simulink model "qpsk_rx_frame_sync"  (R2020a)
settings: Solver=VariableStepAuto  StartTime=0.0  StopTime=4000/3.2e6  RelTol=1e-3
PreLoadFcn:
  | setup_qpsk_receiver
InitFcn:
  | setup_qpsk_receiver
values from neighbouring files (symbols this model uses):
  tx_data = [tx_data mbuf]    [setup_receiver.m]
undefined symbols (not defined in the file or in its folder): AXI4, designMultirateFIR, Lite, xlfda_numerator
libraries: xbsIndex_r4 x244, dspmlti4 x11, hdlsllib x9, dspswit3 x4, commrandsrc3 x2, dspsigops x2, simulink x1
(part 1 of 4)
settings Model: Creator=david  LastModifiedBy=david
settings SFSimCC: CustomCodeUndefinedFunction=UseInterfaceOnly

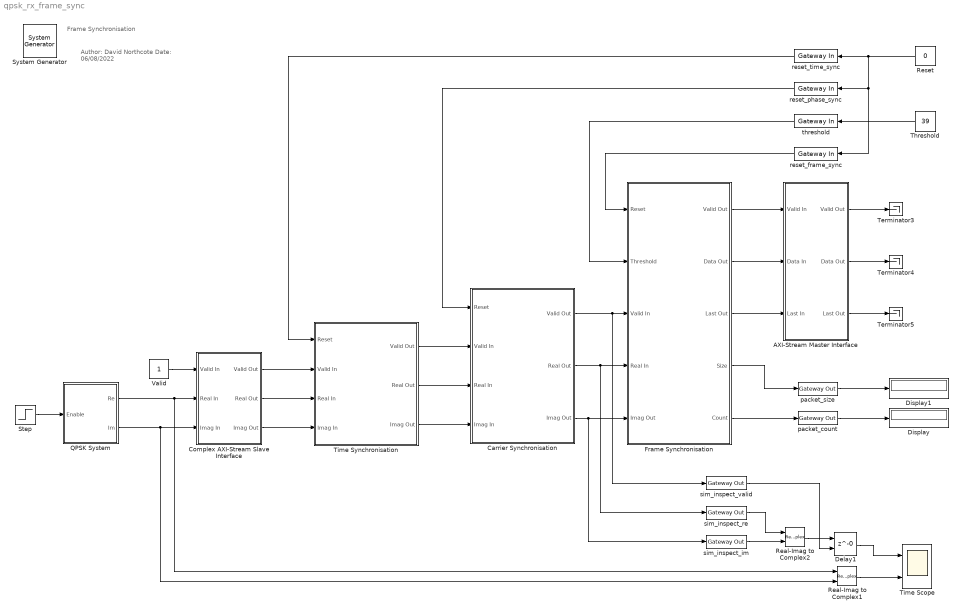
== system qpsk_rx_frame_sync ==
  note: Author: 	David Northcote
      | Date: 	06/08/2022
  note: Frame Synchronisation
  " System Generator" : xbsIndex_r4/ System Generator  Tag=genX  xilinxfamily=zynquplusRFSOC  part=xczu28dr  speed=-2-e  package=ffvg1517  synthesis_tool=Vivado  clock_wrapper=Clock Enables  directory=./netlist  proj_type=Vivado  Synth_file=Vivado Synthesis Defaults  Impl_file=Vivado Implementation Defaults  testbench=off  simulink_period=1/64e6  sysclk_period=(1/64e6)*1e9  dcm_input_clock_period=10  incr_netlist=off  trim_vbits=Everywhere in SubSystem  dbl_ovrd=According to Block Masks  core_generation=According to Block Masks  run_coregen=off  deprecated_control=off  eval_field=0  block_type=sysgen
  AXI-Stream Master Interface : Subsystem
  Carrier Synchronisation : Subsystem
  Complex AXI-Stream Slave Interface : Subsystem
  Delay1 : Delay  DelayLength=0  ShowEnablePort=on
      settings: InputPortMap=u0,e6
  Display : Display
  Display1 : Display
  Frame Synchronisation : Subsystem
  QPSK System : Subsystem
  Real-Imag to Complex1 : RealImagToComplex
  Real-Imag to Complex2 : RealImagToComplex
  Reset : Constant  Value=0  OutDataTypeStr=boolean  SampleTime=-1
  Step : Step  Time=4/12.5e3  SampleTime=1/12.5e3
  Terminator3 : Terminator
  Terminator4 : Terminator
  Terminator5 : Terminator
  Threshold : Constant  Value=39  OutDataTypeStr=uint32  SampleTime=-1
  Time Scope : Scope  NumInputPorts=2
  Time Synchronisation : Subsystem
  Valid : Constant  OutDataTypeStr=boolean  SampleTime=1/3.2e6
  packet_count : xbsIndex_r4/Gateway Out  inherit_from_input=on  hdl_port=on  rows=1  columns=1  UseAsDAC=off  DACChannel='1'  interface=AXI4-Lite  automatic_assignment=off  address_offset=24  intf_name=''  intf_description=''  timing_constraint=None  locs_specified=off  LOCs={}  io_standard={}  block_type=gatewayout
  packet_size : xbsIndex_r4/Gateway Out  inherit_from_input=on  hdl_port=on  rows=1  columns=1  UseAsDAC=off  DACChannel='1'  interface=AXI4-Lite  automatic_assignment=off  address_offset=20  intf_name=''  intf_description=''  timing_constraint=None  locs_specified=off  LOCs={}  io_standard={}  block_type=gatewayout
  reset_frame_sync : xbsIndex_r4/Gateway In  gui_display_data_type=Boolean  arith_type=Boolean  n_bits=16  bin_pt=14  preci_type=Single  exp_width=8  frac_width=24  rows=1  columns=1  quantization="Round  (unbiased: +/- Inf)"  overflow=Saturate  period=1/3.2e6  UseAsADC=off  ADCChannel='1'  interface=AXI4-Lite  automatic_assignment=off  address_offset=8  intf_name=''  intf_description=''  default_value=0  timing_constraint=None  locs_specified=off  LOCs={}  io_standard={}  inherit_from_input=off  hdl_port=on  dbl_ovrd=off  block_type=gatewayin
  reset_phase_sync : xbsIndex_r4/Gateway In  gui_display_data_type=Boolean  arith_type=Boolean  n_bits=16  bin_pt=14  preci_type=Single  exp_width=8  frac_width=24  rows=1  columns=1  quantization="Round  (unbiased: +/- Inf)"  overflow=Saturate  period=1/3.2e6  UseAsADC=off  ADCChannel='1'  interface=AXI4-Lite  automatic_assignment=off  address_offset=4  intf_name=''  intf_description=''  default_value=0  timing_constraint=None  locs_specified=off  LOCs={}  io_standard={}  inherit_from_input=off  hdl_port=on  dbl_ovrd=off  block_type=gatewayin
  reset_time_sync : xbsIndex_r4/Gateway In  gui_display_data_type=Boolean  arith_type=Boolean  n_bits=16  bin_pt=14  preci_type=Single  exp_width=8  frac_width=24  rows=1  columns=1  quantization="Round  (unbiased: +/- Inf)"  overflow=Saturate  period=1/3.2e6  UseAsADC=off  ADCChannel='1'  interface=AXI4-Lite  automatic_assignment=off  address_offset=0  intf_name=''  intf_description=''  default_value=0  timing_constraint=None  locs_specified=off  LOCs={}  io_standard={}  inherit_from_input=off  hdl_port=on  dbl_ovrd=off  block_type=gatewayin
  sim_inspect_im : xbsIndex_r4/Gateway Out  inherit_from_input=on  hdl_port=off  rows=1  columns=1  UseAsDAC=off  DACChannel='1'  interface=None  automatic_assignment=on  address_offset=hex2dec('00')  intf_name=''  intf_description=''  timing_constraint=None  locs_specified=off  LOCs={}  io_standard={}  block_type=gatewayout
  sim_inspect_re : xbsIndex_r4/Gateway Out  inherit_from_input=on  hdl_port=off  rows=1  columns=1  UseAsDAC=off  DACChannel='1'  interface=None  automatic_assignment=on  address_offset=hex2dec('00')  intf_name=''  intf_description=''  timing_constraint=None  locs_specified=off  LOCs={}  io_standard={}  block_type=gatewayout
  sim_inspect_valid : xbsIndex_r4/Gateway Out  inherit_from_input=on  hdl_port=off  rows=1  columns=1  UseAsDAC=off  DACChannel='1'  interface=None  automatic_assignment=on  address_offset=hex2dec('00')  intf_name=''  intf_description=''  timing_constraint=None  locs_specified=off  LOCs={}  io_standard={}  block_type=gatewayout
  threshold : xbsIndex_r4/Gateway In  gui_display_data_type=Fixed-point  arith_type=Unsigned  n_bits=32  bin_pt=0  preci_type=Single  exp_width=8  frac_width=24  rows=1  columns=1  quantization="Round  (unbiased: +/- Inf)"  overflow=Saturate  period=1/3.2e6  UseAsADC=off  ADCChannel='1'  interface=AXI4-Lite  automatic_assignment=off  address_offset=12  intf_name=''  intf_description=''  default_value=0  timing_constraint=None  locs_specified=off  LOCs={}  io_standard={}  inherit_from_input=off  hdl_port=on  dbl_ovrd=off  block_type=gatewayin
  wires:
  QPSK System/1(Re) -> Real-Imag to Complex1/1, Complex AXI-Stream Slave Interface/2(Real In)
  QPSK System/2(Im) -> Real-Imag to Complex1/2, Complex AXI-Stream Slave Interface/3(Imag In)
  Step/1 -> QPSK System/1(Enable)
  Valid/1 -> Complex AXI-Stream Slave Interface/1(Valid In)
  Complex AXI-Stream Slave Interface/1(Valid Out) -> Time Synchronisation/2(Valid In)
  Complex AXI-Stream Slave Interface/2(Real Out) -> Time Synchronisation/3(Real In)
  Complex AXI-Stream Slave Interface/3(Imag Out) -> Time Synchronisation/4(Imag In)
  reset_time_sync/1 -> Time Synchronisation/1(Reset)
  Reset/1 -> reset_phase_sync/1, reset_frame_sync/1, reset_time_sync/1
  Time Synchronisation/1(Valid Out) -> Carrier Synchronisation/2(Valid In)
  Time Synchronisation/2(Real Out) -> Carrier Synchronisation/3(Real In)
  Time Synchronisation/3(Imag Out) -> Carrier Synchronisation/4(Imag In)
  reset_phase_sync/1 -> Carrier Synchronisation/1(Reset)
  Carrier Synchronisation/2(Real Out) -> sim_inspect_re/1, Frame Synchronisation/4(Real In)
  Carrier Synchronisation/1(Valid Out) -> sim_inspect_valid/1, Frame Synchronisation/3(Valid In)
  threshold/1 -> Frame Synchronisation/2(Threshold)
  reset_frame_sync/1 -> Frame Synchronisation/1(Reset)
  Threshold/1 -> threshold/1
  Carrier Synchronisation/3(Imag Out) -> Frame Synchronisation/5(Imag Out), sim_inspect_im/1
  Frame Synchronisation/5(Count) -> packet_count/1
  Frame Synchronisation/4(Size) -> packet_size/1
  AXI-Stream Master Interface/1(Valid Out) -> Terminator3/1
  AXI-Stream Master Interface/2(Data Out) -> Terminator4/1
  AXI-Stream Master Interface/3(Last Out) -> Terminator5/1
  Real-Imag to Complex1/1 -> Time Scope/2
  sim_inspect_valid/1 -> Delay1/2
  Real-Imag to Complex2/1 -> Delay1/1
  sim_inspect_re/1 -> Real-Imag to Complex2/1
  sim_inspect_im/1 -> Real-Imag to Complex2/2
  Delay1/1 -> Time Scope/1
  Frame Synchronisation/1(Valid Out) -> AXI-Stream Master Interface/1(Valid In)
  Frame Synchronisation/2(Data Out) -> AXI-Stream Master Interface/2(Data In)
  Frame Synchronisation/3(Last Out) -> AXI-Stream Master Interface/3(Last In)
  packet_count/1 -> Display/1
  packet_size/1 -> Display1/1

== system qpsk_rx_frame_sync/AXI-Stream Master Interface ==
  note: AXI-Stream
  Valid In : Inport
  Data In : Inport  Port=2
  Last In : Inport  Port=3
  m_axis_tdata : xbsIndex_r4/Gateway Out  inherit_from_input=off  hdl_port=on  rows=1  columns=1  UseAsDAC=off  DACChannel='1'  interface=None  automatic_assignment=on  address_offset=hex2dec('00')  intf_name=''  intf_description=''  timing_constraint=None  locs_specified=off  LOCs={}  io_standard={}  block_type=gatewayout
  m_axis_tlast : xbsIndex_r4/Gateway Out  inherit_from_input=off  hdl_port=on  rows=1  columns=1  UseAsDAC=off  DACChannel='1'  interface=None  automatic_assignment=on  address_offset=hex2dec('00')  intf_name=''  intf_description=''  timing_constraint=None  locs_specified=off  LOCs={}  io_standard={}  block_type=gatewayout
  m_axis_tvalid : xbsIndex_r4/Gateway Out  inherit_from_input=off  hdl_port=on  rows=1  columns=1  UseAsDAC=off  DACChannel='1'  interface=None  automatic_assignment=on  address_offset=hex2dec('00')  intf_name=''  intf_description=''  timing_constraint=None  locs_specified=off  LOCs={}  io_standard={}  block_type=gatewayout
  Valid Out : Outport  VectorParamsAs1DForOutWhenUnconnected=off
  Data Out : Outport  Port=2  VectorParamsAs1DForOutWhenUnconnected=off
  Last Out : Outport  Port=3  VectorParamsAs1DForOutWhenUnconnected=off
  wires:
  Data In/1 -> m_axis_tdata/1
  Valid In/1 -> m_axis_tvalid/1
  m_axis_tdata/1 -> Data Out/1
  m_axis_tvalid/1 -> Valid Out/1
  Last In/1 -> m_axis_tlast/1
  m_axis_tlast/1 -> Last Out/1

== system qpsk_rx_frame_sync/Carrier Synchronisation ==
  Reset : Inport
  Valid In : Inport  Port=2
  Real In : Inport  Port=3
  Imag In : Inport  Port=4
  Convert : xbsIndex_r4/Convert  gui_display_data_type=Fixed-point  arith_type="Signed  (2's comp)"  n_bits=16  bin_pt=14  float_type=Single  exp_bits=8  fraction_bits=24  quantization=Truncate  overflow=Wrap  en=off  latency=0  pipeline=off  dbl_ovrd=off  block_type=convert
  Convert1 : xbsIndex_r4/Convert  gui_display_data_type=Fixed-point  arith_type="Signed  (2's comp)"  n_bits=16  bin_pt=14  float_type=Single  exp_bits=8  fraction_bits=24  quantization=Truncate  overflow=Wrap  en=off  latency=0  pipeline=off  dbl_ovrd=off  block_type=convert
  De-Rotate Constellation : Subsystem
  Generate Angle Error : Subsystem
  Generate NCO : Subsystem
  Valid Out : Outport  VectorParamsAs1DForOutWhenUnconnected=off
  Real Out : Outport  Port=2  VectorParamsAs1DForOutWhenUnconnected=off
  Imag Out : Outport  Port=3  VectorParamsAs1DForOutWhenUnconnected=off
  wires:
  Reset/1 -> Generate NCO/3(Reset)
  De-Rotate Constellation/1(Imag Out) -> Convert/1
  De-Rotate Constellation/2(Real Out) -> Convert1/1
  De-Rotate Constellation/3(Valid Out) -> Valid Out/1, Generate Angle Error/3(Valid In)
  Generate NCO/3(Valid Out) -> De-Rotate Constellation/6(Valid Error)
  Generate NCO/2(Real Out) -> De-Rotate Constellation/5(Real Error)
  Generate NCO/1(Imag Out) -> De-Rotate Constellation/4(Imag Error)
  Generate Angle Error/1(Angle) -> Generate NCO/1(Angle)
  Generate Angle Error/2(Valid Out) -> Generate NCO/2(Valid In)
  Valid In/1 -> De-Rotate Constellation/3(Valid In)
  Real In/1 -> De-Rotate Constellation/2(Real In)
  Imag In/1 -> De-Rotate Constellation/1(Imag In)
  Convert/1 -> Imag Out/1, Generate Angle Error/1(Imag In)
  Convert1/1 -> Real Out/1, Generate Angle Error/2(Real In)

== system qpsk_rx_frame_sync/Complex AXI-Stream Slave Interface ==
  note: AXI-Stream Real
  note: AXI-Stream Imag
  Valid In : Inport
  Real In : Inport  Port=2
  Imag In : Inport  Port=3
  Terminator : Terminator
  s_axis_tdata_im : xbsIndex_r4/Gateway In  gui_display_data_type=Fixed-point  arith_type="Signed  (2's comp)"  n_bits=16  bin_pt=14  preci_type=Single  exp_width=8  frac_width=24  rows=1  columns=1  quantization="Round  (unbiased: +/- Inf)"  overflow=Saturate  period=1/3.2e6  UseAsADC=off  ADCChannel='1'  interface=None  automatic_assignment=on  address_offset=hex2dec('00')  intf_name=''  intf_description=''  default_value=0  timing_constraint=None  locs_specified=off  LOCs={}  io_standard={}  inherit_from_input=off  hdl_port=on  dbl_ovrd=off  block_type=gatewayin
  s_axis_tdata_re : xbsIndex_r4/Gateway In  gui_display_data_type=Fixed-point  arith_type="Signed  (2's comp)"  n_bits=16  bin_pt=14  preci_type=Single  exp_width=8  frac_width=24  rows=1  columns=1  quantization="Round  (unbiased: +/- Inf)"  overflow=Saturate  period=1/3.2e6  UseAsADC=off  ADCChannel='1'  interface=None  automatic_assignment=on  address_offset=hex2dec('00')  intf_name=''  intf_description=''  default_value=0  timing_constraint=None  locs_specified=off  LOCs={}  io_standard={}  inherit_from_input=off  hdl_port=on  dbl_ovrd=off  block_type=gatewayin
  s_axis_tvalid_im : xbsIndex_r4/Gateway In  gui_display_data_type=Boolean  arith_type=Boolean  n_bits=16  bin_pt=14  preci_type=Single  exp_width=8  frac_width=24  rows=1  columns=1  quantization="Round  (unbiased: +/- Inf)"  overflow=Saturate  period=1/3.2e6  UseAsADC=off  ADCChannel='1'  interface=None  automatic_assignment=on  address_offset=hex2dec('00')  intf_name=''  intf_description=''  default_value=0  timing_constraint=None  locs_specified=off  LOCs={}  io_standard={}  inherit_from_input=off  hdl_port=on  dbl_ovrd=off  block_type=gatewayin
  s_axis_tvalid_re : xbsIndex_r4/Gateway In  gui_display_data_type=Boolean  arith_type=Boolean  n_bits=16  bin_pt=14  preci_type=Single  exp_width=8  frac_width=24  rows=1  columns=1  quantization="Round  (unbiased: +/- Inf)"  overflow=Saturate  period=1/3.2e6  UseAsADC=off  ADCChannel='1'  interface=None  automatic_assignment=on  address_offset=hex2dec('00')  intf_name=''  intf_description=''  default_value=0  timing_constraint=None  locs_specified=off  LOCs={}  io_standard={}  inherit_from_input=off  hdl_port=on  dbl_ovrd=off  block_type=gatewayin
  Valid Out : Outport  VectorParamsAs1DForOutWhenUnconnected=off
  Real Out : Outport  Port=2  VectorParamsAs1DForOutWhenUnconnected=off
  Imag Out : Outport  Port=3  VectorParamsAs1DForOutWhenUnconnected=off
  wires:
  Imag In/1 -> s_axis_tdata_im/1
  s_axis_tdata_re/1 -> Real Out/1
  s_axis_tdata_im/1 -> Imag Out/1
  Valid In/1 -> s_axis_tvalid_im/1, s_axis_tvalid_re/1
  s_axis_tvalid_re/1 -> Valid Out/1
  s_axis_tvalid_im/1 -> Terminator/1
  Real In/1 -> s_axis_tdata_re/1

== system qpsk_rx_frame_sync/Frame Synchronisation ==
  Reset : Inport
  Threshold : Inport  Port=2
  Valid In : Inport  Port=3
  Real In : Inport  Port=4
  Imag Out : Inport  Port=5
  Convert to AXI-Stream : Subsystem
  Frame Sync : Subsystem
  Valid Out : Outport  VectorParamsAs1DForOutWhenUnconnected=off
  Data Out : Outport  Port=2  VectorParamsAs1DForOutWhenUnconnected=off
  Last Out : Outport  Port=3  VectorParamsAs1DForOutWhenUnconnected=off
  Size : Outport  Port=4  VectorParamsAs1DForOutWhenUnconnected=off
  Count : Outport  Port=5  VectorParamsAs1DForOutWhenUnconnected=off
  wires:
  Convert to AXI-Stream/4(Size) -> Size/1
  Frame Sync/3(count) -> Count/1
  Convert to AXI-Stream/5(Reset) -> Frame Sync/6(Reset)
  Convert to AXI-Stream/3(Last Out) -> Last Out/1
  Convert to AXI-Stream/2(Valid Out) -> Valid Out/1
  Convert to AXI-Stream/1(Data Out) -> Data Out/1
  Frame Sync/2(Valid Out) -> Convert to AXI-Stream/2(Valid In)
  Frame Sync/1(Data Out) -> Convert to AXI-Stream/1(Data In)
  Reset/1 -> Frame Sync/5(reset_count)
  Valid In/1 -> Frame Sync/4(Valid In)
  Real In/1 -> Frame Sync/2(Real)
  Threshold/1 -> Frame Sync/1(Threshold)
  Imag Out/1 -> Frame Sync/3(Imag)

== system qpsk_rx_frame_sync/QPSK System ==
  Enable : Inport
  Complex to Real-Imag : ComplexToRealImag
  QPSK RX Generation : Subsystem
  QPSK TX Generation : Subsystem
  RF Balun Gain RX : Gain  Gain=1/2
  RF Balun Gain TX : Gain  Gain=1/2
  RF-ADC : Subsystem  mask{fs_ghz=1.024, decim=8x, ssr=2, mode=Fine, fc=0.064, fph=0, fcoarse=fs/4}
      mask prompts: fs_ghz "Sample Rate (GHz):"; decim "Interpolation Mode:"; ssr "Samples per AXI4-Stream Cycle:"; mode "Mixer Type:"; fc "NCO Frequency (GHz):"; fph "NCO Phase (Rads):"; fcoarse "Frequency:"
      mask init:
      | % Obtain the sample rate in Hz
      | fs = str2double(get_param(gcb, 'fs_ghz'))*1e9;
      | 
      | % Set the mode of the RF-DAC interpolation filter
      | switch get_param(gcb, 'decim')
      |     case '1x'
      |         D = 1;
      |     case '2x'
      |         D = 2;
      |     case '4x'
      |         D = 4;
      |     case '8x'
      |         D = 8;
      |     otherwise
      |         D = 1;
      | end
      | 
      | % Get the AXI-Stream clock for display to user
      | axi_clk = (fs/(str2double(get_param(gcb, 'ssr'))*D))*1e-6;
      | 
      | % Get the block mask object to manipulate settings
      | mo = get_param(gcb, 'MaskObject');
      | 
      | % Update text to display the required AXI-Stream clock
      | tc = mo.getDialogControl('axi_text');
      | tc.Prompt = ['      Required AXI-Stream Clock: ', num2str(axi_clk), ' MHz'];
      | 
      | % Set the RF-DAC Mixer mode
      | switch get_param(gcb, 'mode')
      |     case 'Bypass'
      |         m = 0;
      |     case 'Coarse'
      |         m = 1;
      |     case 'Fine'
      |         m = 2;
      |     otherwise
      |         m = 0;
      | end
      | 
      | % Set the RF-DAC Coarse Mixer mode
      | switch get_param(gcb, 'fcoarse')
      |     case 'fs/2'
      |         mc = 0;
      |     case 'fs/4'
      |         mc = 1;
      |     case '-fs/4'
      |         mc = 2;
      |     otherwise
      |         mc = 0;
      | end
      | 
      | % Set other blocks
      | set_param([gcb, '/Decimation Filter'], 'decim', get_param(gcb, 'decim'));
      mask Callback fs_ghz:
      | % Obtain the sample rate in Hz
      | fs = str2double(get_param(gcb, 'fs_ghz'))*1e9;
      | 
      | % Set the mode of the RF-DAC interpolation filter
      | switch get_param(gcb, 'decim')
      |     case '1x'
      |         D = 1;
      |     case '2x'
      |         D = 2;
      |     case '4x'
      |         D = 4;
      |     case '8x'
      |         D = 8;
      |     otherwise
      |         D = 1;
      | end
      | 
      | % Get the AXI-Stream clock for display to user
      | axi_clk = (fs/(str2double(get_param(gcb, 'ssr'))*D))*1e-6;
      | 
      | % Get the block mask object to manipulate settings
      | mo = get_param(gcb, 'MaskObject');
      | 
      | % Update text to display the required AXI-Stream clock
      | tc = mo.getDialogControl('axi_text');
      | tc.Prompt = ['      Required AXI-Stream Clock: ', num2str(axi_clk), ' MHz'];
      mask TypeOptions decim: 1x | 2x | 4x | 8x
      mask Callback decim:
      | % Obtain the sample rate in Hz
      | fs = str2double(get_param(gcb, 'fs_ghz'))*1e9;
      | 
      | % Set the mode of the RF-DAC interpolation filter
      | switch get_param(gcb, 'decim')
      |     case '1x'
      |         D = 1;
      |     case '2x'
      |         D = 2;
      |     case '4x'
      |         D = 4;
      |     case '8x'
      |         D = 8;
      |     otherwise
      |         D = 1;
      | end
      | 
      | % Get the AXI-Stream clock for display to user
      | axi_clk = (fs/(str2double(get_param(gcb, 'ssr'))*D))*1e-6;
      | 
      | % Get the block mask object to manipulate settings
      | mo = get_param(gcb, 'MaskObject');
      | 
      | % Update text to display the required AXI-Stream clock
      | tc = mo.getDialogControl('axi_text');
      | tc.Prompt = ['      Required AXI-Stream Clock: ', num2str(axi_clk), ' MHz'];
      mask TypeOptions ssr: 1 | 2 | 3 | 4 | 5 | 6 | 7 | 8 | 9 | 10 | 11 | 12 | 13 | 14 | 15 | 16
      mask Callback ssr:
      | % Obtain the sample rate in Hz
      | fs = str2double(get_param(gcb, 'fs_ghz'))*1e9;
      | 
      | % Set the mode of the RF-DAC interpolation filter
      | switch get_param(gcb, 'decim')
      |     case '1x'
      |         D = 1;
      |     case '2x'
      |         D = 2;
      |     case '4x'
      |         D = 4;
      |     case '8x'
      |         D = 8;
      |     otherwise
      |         D = 1;
      | end
      | 
      | % Get the AXI-Stream clock for display to user
      | axi_clk = (fs/(str2double(get_param(gcb, 'ssr'))*D))*1e-6;
      | 
      | % Get the block mask object to manipulate settings
      | mo = get_param(gcb, 'MaskObject');
      | 
      | % Update text to display the required AXI-Stream clock
      | tc = mo.getDialogControl('axi_text');
      | tc.Prompt = ['      Required AXI-Stream Clock: ', num2str(axi_clk), ' MHz'];
      mask TypeOptions mode: Coarse | Fine
      mask Callback mode:
      | % Get the block mask object to manipulate settings
      | mo = get_param(gcb, 'MaskObject');
      | 
      | % Hide group depending on Mixer mode choice
      | switch get_param(gcb, 'mode')
      |     case 'Bypass'
      |         mo.getDialogControl('coarse_group').Visible='off';
      |         mo.getDialogControl('mixer_group').Visible='off';
      |     case 'Coarse'
      |         mo.getDialogControl('coarse_group').Visible='on';
      |         mo.getDialogControl('mixer_group').Visible='off';
      |     case 'Fine'
      |         mo.getDialogControl('coarse_group').Visible='off';
      |         mo.getDialogControl('mixer_group').Visible='on';
      |     otherwise
      |         mo.getDialogControl('coarse_group').Visible='off';
      |         mo.getDialogControl('mixer_group').Visible='off';
      | end
      mask TypeOptions fcoarse: fs/2 | fs/4 | -fs/4
      mask DialogControl DescGroupVar Prompt: RF-DAC
      mask DialogControl DescTextVar Prompt: This block simulates one RF-ADC channel.
      mask DialogControl main_group Prompt: Data Settings
      mask DialogControl axi_text Prompt: Required AXI-Stream Clock: 64 MHz
      mask DialogControl Container5 Prompt: Mixer Settings
  RF-DAC : Subsystem  mask{fs_ghz=1.024, interp=8x, ssr=1, mode=Fine, fc=0.064, fph=0, fcoarse=fs/4}
      mask prompts: fs_ghz "Sample Rate (GHz):"; interp "Interpolation Mode:"; ssr "Samples per AXI4-Stream Cycle:"; mode "Mixer Type:"; fc "NCO Frequency (GHz):"; fph "NCO Phase (Rads):"; fcoarse "Frequency:"
      mask init:
      | % Obtain the sample rate in Hz
      | fs = str2double(get_param(gcb, 'fs_ghz'))*1e9;
      | 
      | % Set the mode of the RF-DAC interpolation filter
      | switch get_param(gcb, 'interp')
      |     case '1x'
      |         L = 1;
      |     case '2x'
      |         L = 2;
      |     case '4x'
      |         L = 4;
      |     case '8x'
      |         L = 8;
      |     otherwise
      |         L = 1;
      | end
      | 
      | % Get the AXI-Stream clock for display to user
      | axi_clk = (fs/(str2double(get_param(gcb, 'ssr'))*L))*1e-6;
      | 
      | % Get the block mask object to manipulate settings
      | mo = get_param(gcb, 'MaskObject');
      | 
      | % Update text to display the required AXI-Stream clock
      | tc = mo.getDialogControl('axi_text');
      | tc.Prompt = ['      Required AXI-Stream Clock: ', num2str(axi_clk), ' MHz'];
      | 
      | % Set the RF-DAC Mixer mode
      | switch get_param(gcb, 'mode')
      |     case 'Bypass'
      |         m = 0;
      |     case 'Coarse'
      |         m = 1;
      |     case 'Fine'
      |         m = 2;
      |     otherwise
      |         m = 0;
      | end
      | 
      | % Set the RF-DAC Coarse Mixer mode
      | switch get_param(gcb, 'fcoarse')
      |     case 'fs/2'
      |         mc = 0;
      |     case 'fs/4'
      |         mc = 1;
      |     case '-fs/4'
      |         mc = 2;
      |     otherwise
      |         mc = 0;
      | end
      | 
      | % Set other blocks
      | set_param([gcb, '/Interpolation Filter'], 'interp', get_param(gcb, 'interp'));
      mask Callback fs_ghz:
      | % Obtain the sample rate in Hz
      | fs = str2double(get_param(gcb, 'fs_ghz'))*1e9;
      | 
      | % Set the mode of the RF-DAC interpolation filter
      | switch get_param(gcb, 'interp')
      |     case '1x'
      |         L = 1;
      |     case '2x'
      |         L = 2;
      |     case '4x'
      |         L = 4;
      |     case '8x'
      |         L = 8;
      |     otherwise
      |         L = 1;
      | end
      | 
      | % Get the AXI-Stream clock for display to user
      | axi_clk = (fs/(str2double(get_param(gcb, 'ssr'))*L))*1e-6;
      | 
      | % Get the block mask object to manipulate settings
      | mo = get_param(gcb, 'MaskObject');
      | 
      | % Update text to display the required AXI-Stream clock
      | tc = mo.getDialogControl('axi_text');
      | tc.Prompt = ['      Required AXI-Stream Clock: ', num2str(axi_clk), ' MHz'];
      mask TypeOptions interp: 1x | 2x | 4x | 8x
      mask Callback interp:
      | % Obtain the sample rate in Hz
      | fs = str2double(get_param(gcb, 'fs_ghz'))*1e9;
      | 
      | % Set the mode of the RF-DAC interpolation filter
      | switch get_param(gcb, 'interp')
      |     case '1x'
      |         L = 1;
      |     case '2x'
      |         L = 2;
      |     case '4x'
      |         L = 4;
      |     case '8x'
      |         L = 8;
      |     otherwise
      |         L = 1;
      | end
      | 
      | % Get the AXI-Stream clock for display to user
      | axi_clk = (fs/(str2double(get_param(gcb, 'ssr'))*L))*1e-6;
      | 
      | % Get the block mask object to manipulate settings
      | mo = get_param(gcb, 'MaskObject');
      | 
      | % Update text to display the required AXI-Stream clock
      | tc = mo.getDialogControl('axi_text');
      | tc.Prompt = ['      Required AXI-Stream Clock: ', num2str(axi_clk), ' MHz'];
      mask TypeOptions ssr: 1 | 2 | 3 | 4 | 5 | 6 | 7 | 8 | 9 | 10 | 11 | 12 | 13 | 14 | 15 | 16
      mask Callback ssr:
      | % Obtain the sample rate in Hz
      | fs = str2double(get_param(gcb, 'fs_ghz'))*1e9;
      | 
      | % Set the mode of the RF-DAC interpolation filter
      | switch get_param(gcb, 'interp')
      |     case '1x'
      |         L = 1;
      |     case '2x'
      |         L = 2;
      |     case '4x'
      |         L = 4;
      |     case '8x'
      |         L = 8;
      |     otherwise
      |         L = 1;
      | end
      | 
      | % Get the AXI-Stream clock for display to user
      | axi_clk = (fs/(str2double(get_param(gcb, 'ssr'))*L))*1e-6;
      | 
      | % Get the block mask object to manipulate settings
      | mo = get_param(gcb, 'MaskObject');
      | 
      | % Update text to display the required AXI-Stream clock
      | tc = mo.getDialogControl('axi_text');
      | tc.Prompt = ['      Required AXI-Stream Clock: ', num2str(axi_clk), ' MHz'];
      mask TypeOptions mode: Coarse | Fine
      mask Callback mode:
      | % Get the block mask object to manipulate settings
      | mo = get_param(gcb, 'MaskObject');
      | 
      | % Hide group depending on Mixer mode choice
      | switch get_param(gcb, 'mode')
      |     case 'Bypass'
      |         mo.getDialogControl('coarse_group').Visible='off';
      |         mo.getDialogControl('mixer_group').Visible='off';
      |     case 'Coarse'
      |         mo.getDialogControl('coarse_group').Visible='on';
      |         mo.getDialogControl('mixer_group').Visible='off';
      |     case 'Fine'
      |         mo.getDialogControl('coarse_group').Visible='off';
      |         mo.getDialogControl('mixer_group').Visible='on';
      |     otherwise
      |         mo.getDialogControl('coarse_group').Visible='off';
      |         mo.getDialogControl('mixer_group').Visible='off';
      | end
      mask TypeOptions fcoarse: fs/2 | fs/4 | -fs/4
      mask DialogControl DescGroupVar Prompt: RF-DAC
      mask DialogControl DescTextVar Prompt: This block simulates one RF-DAC channel.
      mask DialogControl main_group Prompt: Data Settings
      mask DialogControl axi_text Prompt: Required AXI-Stream Clock: 128 MHz
      mask DialogControl Container5 Prompt: Mixer Settings
  Re : Outport  VectorParamsAs1DForOutWhenUnconnected=off
  Im : Outport  Port=2  VectorParamsAs1DForOutWhenUnconnected=off
  wires:
  Enable/1 -> QPSK TX Generation/1(Enable)
  Complex to Real-Imag/1 -> Re/1
  Complex to Real-Imag/2 -> Im/1
  RF-DAC/1(Data Out) -> RF Balun Gain TX/1
  RF Balun Gain TX/1 -> RF Balun Gain RX/1
  RF Balun Gain RX/1 -> RF-ADC/1(Data In)
  QPSK TX Generation/1(QPSK) -> RF-DAC/1(Data In)
  QPSK RX Generation/1(Data Out) -> Complex to Real-Imag/1
  RF-ADC/1(Data Out) -> QPSK RX Generation/1(Data In)

== system qpsk_rx_frame_sync/Time Synchronisation ==
  Reset : Inport
  Valid In : Inport  Port=2
  Real In : Inport  Port=3
  Imag In : Inport  Port=4
  Loop Filter : Subsystem  mask{T=1/100e3, d=1/sqrt(2), Kp=1/sqrt(2), Bn=0.07071*100e3, Ko=1}
      mask prompts: T "Sampling Period:"; d "Damping Ratio:"; Kp "Phase Detector Gain:"; Bn "Noise Bandwidth:"; Ko "Oscillator Gain:"
      mask init:
      | n = (Bn*T)/(d+1/(4*d));
      | 
      | K1 = ((4*d*n)/(1+2*d*n+n^2))/(Ko*Kp);
      | 
      | K2 = ((4*n^2)/(1+2*d*n+n^2))/(Ko*Kp);
      | 
      | %K1 = (4*d*n)/(Ko*Kp);
      | 
      | %K2 = (4*(n^2))/(Ko*Kp);
      mask DialogControl DescGroupVar Prompt: Loop Filter
      mask DialogControl DescTextVar Prompt: A simplified loop filter.
      mask DialogControl ParameterGroupVar Prompt: Main
  NCC : Subsystem  mask{r=32}
      mask prompts: r "Symbol Oversample Factor:"
      mask init:
      | n = ceil(log2(r));
      | f = 32-n;
      mask DialogControl DescGroupVar Prompt: Numerically Controlled Clock (NCC)
      mask DialogControl DescTextVar Prompt: The NCC block contains an accumulator that increments by one each clock cycle. The wordlength of the accumulator is determined by the symbol oversampling factor. Once the maximum value of the accumulator is reached, the accumulation starts again. The error signal can be used to increase or decrease the rate of accumulation. When the accumulator wraps around, a binary high is released from the strobe port.
      mask DialogControl ParameterGroupVar Prompt: Main
  Terminator : Terminator
  Timing Error Detector : Subsystem
  Valid Out : Outport  VectorParamsAs1DForOutWhenUnconnected=off
  Real Out : Outport  Port=2  VectorParamsAs1DForOutWhenUnconnected=off
  Imag Out : Outport  Port=3  VectorParamsAs1DForOutWhenUnconnected=off
  wires:
  Reset/1 -> Loop Filter/5(Reset)
  NCC/1(Strobe) -> Loop Filter/4(Valid In)
  Loop Filter/2(Imag Out) -> Imag Out/1
  Loop Filter/1(Real Out) -> Real Out/1
  Loop Filter/3(Valid Out) -> Valid Out/1
  Imag In/1 -> Timing Error Detector/2(Imag In), Loop Filter/2(Imag In)
  Timing Error Detector/1(Error) -> Loop Filter/3(Signal In)
  Loop Filter/4(Error Out) -> NCC/1(Error)
  Real In/1 -> Loop Filter/1(Real In), Timing Error Detector/1(Real In)
  Valid In/1 -> Terminator/1

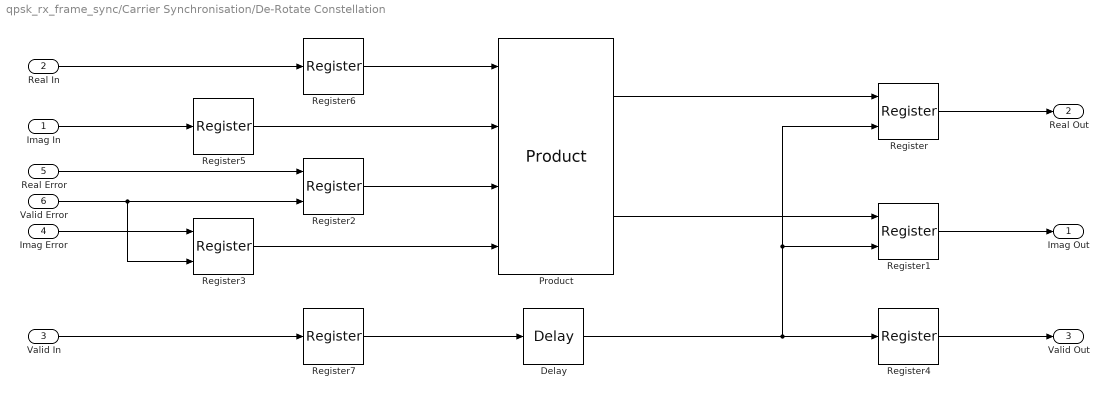
== system qpsk_rx_frame_sync/Carrier Synchronisation/De-Rotate Constellation ==
  Imag In : Inport
  Real In : Inport  Port=2
  Valid In : Inport  Port=3
  Imag Error : Inport  Port=4
  Real Error : Inport  Port=5
  Valid Error : Inport  Port=6
  Delay : xbsIndex_r4/Delay  rst=off  infoeditControl=Selection of Reset will increase slice count due to use of real FFs and instead of SRLs  en=off  latency=4  reg_retiming=off  dbl_ovrd=off  block_type=delay
  Product : xbsIndex_r4/Product  complex_multiplier=on  optimizegoal=Performance  simulation_type=fast_sim  simulation_model=sysgen:product_macro  block_type=product_macro
  Register{,1..3} (4 alike) : xbsIndex_r4/Register  init=0  rst=off  en=on  dbl_ovrd=off  block_type=register
  Register{4..7} (4 alike) : xbsIndex_r4/Register  init=0  rst=off  en=off  dbl_ovrd=off  block_type=register
  Imag Out : Outport  VectorParamsAs1DForOutWhenUnconnected=off
  Real Out : Outport  Port=2  VectorParamsAs1DForOutWhenUnconnected=off
  Valid Out : Outport  Port=3  VectorParamsAs1DForOutWhenUnconnected=off
  wires:
  Register/1 -> Real Out/1
  Register1/1 -> Imag Out/1
  Valid In/1 -> Register7/1
  Imag Error/1 -> Register3/1
  Register4/1 -> Valid Out/1
  Register7/1 -> Delay/1
  Real Error/1 -> Register2/1
  Imag In/1 -> Register5/1
  Real In/1 -> Register6/1
  Valid Error/1 -> Register3/2, Register2/2
  Delay/1 -> Register/2, Register1/2, Register4/1
  Register6/1 -> Product/1
  Register5/1 -> Product/2
  Register2/1 -> Product/3
  Register3/1 -> Product/4
  Product/1 -> Register/1
  Product/2 -> Register1/1

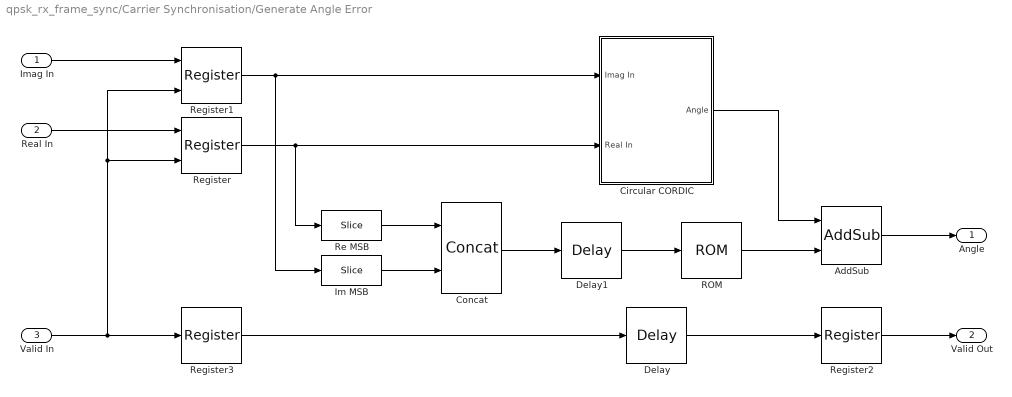
== system qpsk_rx_frame_sync/Carrier Synchronisation/Generate Angle Error ==
  Imag In : Inport
  Real In : Inport  Port=2
  Valid In : Inport  Port=3
  AddSub : xbsIndex_r4/AddSub  mode=Subtraction  use_carryin=off  use_carryout=off  en=off  latency=1  precision=Full  arith_type=Unsigned  n_bits=16  bin_pt=14  quantization=Truncate  overflow=Wrap  use_behavioral_HDL=off  hw_selection=Fabric  pipelined=off  dbl_ovrd=off  block_type=addsub
  Circular CORDIC : Subsystem
  Concat : xbsIndex_r4/Concat  num_inputs=2  dbl_ovrd=off  block_type=concat
  Delay : xbsIndex_r4/Delay  rst=off  infoeditControl=Selection of Reset will increase slice count due to use of real FFs and instead of SRLs  en=off  latency=8  reg_retiming=off  dbl_ovrd=off  block_type=delay
  Delay1 : xbsIndex_r4/Delay  rst=off  infoeditControl=Selection of Reset will increase slice count due to use of real FFs and instead of SRLs  en=off  latency=7  reg_retiming=off  dbl_ovrd=off  block_type=delay
  Im MSB : xbsIndex_r4/Slice  nbits=1  boolean_output=off  mode=Upper Bit Location + Width  bit1=0  base1=MSB of Input  bit0=0  base0=LSB of Input  dbl_ovrd=off  block_type=slice
  ROM : xbsIndex_r4/ROM  depth=4  initVector=[pi/4 -pi/4 -pi/4 pi/4]  distributed_mem=Block RAM  rst=off  init_reg=0  en=off  latency=1  gui_display_data_type=Fixed-point  arith_type="Signed  (2's comp)"  n_bits=16  bin_pt=14  preci_type=Single  exp_width=8  frac_width=24  optimize=Area  use_rpm=on  dbl_ovrd=off  simulation_type=fast_sim  block_type=sprom
  Re MSB : xbsIndex_r4/Slice  nbits=1  boolean_output=off  mode=Upper Bit Location + Width  bit1=0  base1=MSB of Input  bit0=0  base0=LSB of Input  dbl_ovrd=off  block_type=slice
  Register : xbsIndex_r4/Register  init=0  rst=off  en=on  dbl_ovrd=off  block_type=register
  Register1 : xbsIndex_r4/Register  init=0  rst=off  en=on  dbl_ovrd=off  block_type=register
  Register2 : xbsIndex_r4/Register  init=0  rst=off  en=off  dbl_ovrd=off  block_type=register
  Register3 : xbsIndex_r4/Register  init=0  rst=off  en=off  dbl_ovrd=off  block_type=register
  Angle : Outport  VectorParamsAs1DForOutWhenUnconnected=off
  Valid Out : Outport  Port=2  VectorParamsAs1DForOutWhenUnconnected=off
  wires:
  Valid In/1 -> Register3/1, Register/2, Register1/2
  Real In/1 -> Register/1
  Imag In/1 -> Register1/1
  Register1/1 -> Im MSB/1, Circular CORDIC/1(Imag In)
  Register3/1 -> Delay/1
  Register/1 -> Re MSB/1, Circular CORDIC/2(Real In)
  Re MSB/1 -> Concat/1
  Im MSB/1 -> Concat/2
  Concat/1 -> Delay1/1
  Delay1/1 -> ROM/1
  AddSub/1 -> Angle/1
  ROM/1 -> AddSub/2
  Circular CORDIC/1(Angle) -> AddSub/1
  Delay/1 -> Register2/1
  Register2/1 -> Valid Out/1

== system qpsk_rx_frame_sync/Carrier Synchronisation/Generate NCO ==
  Angle : Inport
  Valid In : Inport  Port=2
  Reset : Inport  Port=3
  Loop Filter : Subsystem  mask{T=1/(100e3*32), d=0.707, Kp=1, Bn=0.04*(100e3*32), Ko=1}
      mask prompts: T "Sampling Period:"; d "Damping Ratio:"; Kp "Phase Detector Gain:"; Bn "Noise Bandwidth:"; Ko "Oscillator Gain:"
      mask init:
      | n = (Bn*T)/(d+1/(4*d));
      | 
      | %K1 = ((4*d*n)/(1+2*d*n+n^2))/(Ko*Kp);
      | 
      | %K2 = ((4*n^2)/(1+2*d*n+n^2))/(Ko*Kp);
      | 
      | K1 = (4*d*n)/(Ko*Kp);
      | 
      | K2 = (4*(n^2))/(Ko*Kp);
  NCO : Subsystem  mask(NCO){n=8, b=34}
      mask prompts: n "Number of integer_bits"; b "Number of fractional bits"
      mask help:
      | Numerically Controller Oscillator.
      |
      | Integrates the phase error and generates cosine and negative sign outputs.
      mask init:
      | k_n = ceil(log2((2^n)/(2*pi)));
      mask DialogControl Container3 Prompt: Accumulator
  Imag Out : Outport  VectorParamsAs1DForOutWhenUnconnected=off
  Real Out : Outport  Port=2  VectorParamsAs1DForOutWhenUnconnected=off
  Valid Out : Outport  Port=3  VectorParamsAs1DForOutWhenUnconnected=off
  wires:
  Reset/1 -> Loop Filter/3(Reset)
  NCO/1(Cos) -> Real Out/1
  NCO/2(Neg Sin) -> Imag Out/1
  Loop Filter/2(Valid) -> NCO/2(En_in)
  Loop Filter/1(Error) -> NCO/1(Step Size)
  Valid In/1 -> Loop Filter/2(Strobe)
  Angle/1 -> Loop Filter/1(Signal)
  NCO/3(En_out) -> Valid Out/1

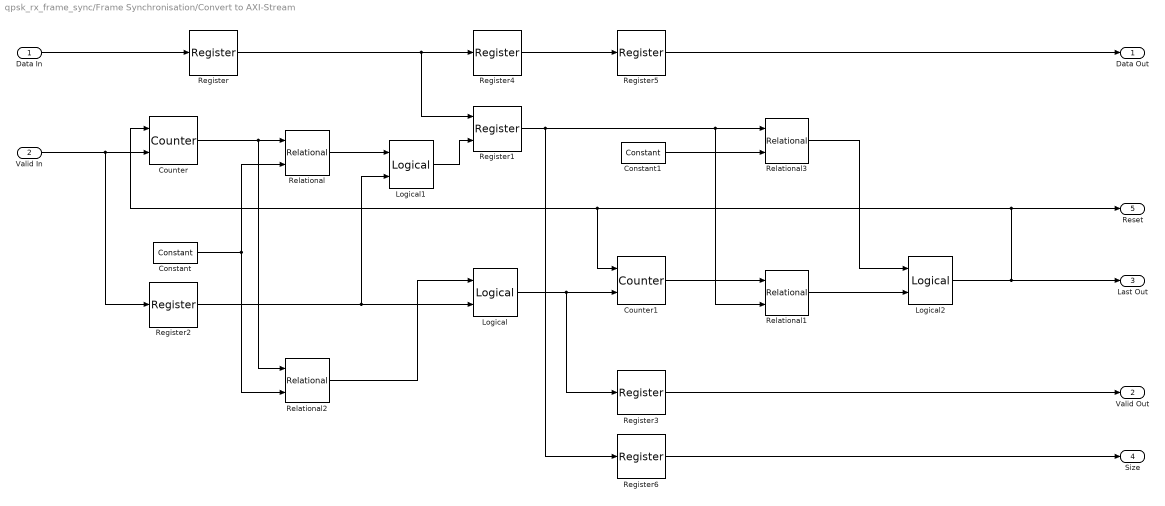
== system qpsk_rx_frame_sync/Frame Synchronisation/Convert to AXI-Stream ==
  Data In : Inport
  Valid In : Inport  Port=2
  Constant : xbsIndex_r4/Constant  const=1.0  gui_display_data_type=Fixed-point  arith_type=Unsigned  n_bits=1  bin_pt=0  preci_type=Single  exp_width=8  frac_width=24  explicit_period=off  period=1  equ=P=C  opselect=C  inp2=PCIN>>17  opr=+  inp1=P  carry=CIN  dbl_ovrd=off  block_type=constant
  Constant1 : xbsIndex_r4/Constant  const=0  gui_display_data_type=Fixed-point  arith_type=Unsigned  n_bits=1  bin_pt=0  preci_type=Single  exp_width=8  frac_width=24  explicit_period=off  period=1  equ=P=C  opselect=C  inp2=PCIN>>17  opr=+  inp1=P  carry=CIN  dbl_ovrd=off  block_type=constant
  Counter : xbsIndex_r4/Counter  cnt_type=Free Running  cnt_to=Inf  operation=Up  start_count=0  cnt_by_val=1  arith_type=Unsigned  n_bits=32  bin_pt=0  load_pin=off  rst=on  en=on  explicit_period=off  period=1  use_behavioral_HDL=off  implementation=Fabric  dbl_ovrd=off  block_type=counter
  Counter1 : xbsIndex_r4/Counter  cnt_type=Free Running  cnt_to=Inf  operation=Up  start_count=0  cnt_by_val=1  arith_type=Unsigned  n_bits=32  bin_pt=0  load_pin=off  rst=on  en=on  explicit_period=off  period=1  use_behavioral_HDL=off  implementation=Fabric  dbl_ovrd=off  block_type=counter
  Logical : xbsIndex_r4/Logical  logical_function=AND  inputs=2  en=off  latency=1  precision=Full  arith_type=Unsigned  n_bits=16  bin_pt=0  align_bp=on  dbl_ovrd=off  block_type=logical
  Logical1 : xbsIndex_r4/Logical  logical_function=AND  inputs=2  en=off  latency=0  precision=Full  arith_type=Unsigned  n_bits=16  bin_pt=0  align_bp=on  dbl_ovrd=off  block_type=logical
  Logical2 : xbsIndex_r4/Logical  logical_function=AND  inputs=2  en=off  latency=0  precision=Full  arith_type=Unsigned  n_bits=16  bin_pt=0  align_bp=on  dbl_ovrd=off  block_type=logical
  Register{,2..6} (6 alike) : xbsIndex_r4/Register  init=0  rst=off  en=off  dbl_ovrd=off  block_type=register
  Register1 : xbsIndex_r4/Register  init=0  rst=off  en=on  dbl_ovrd=off  block_type=register
  Relational : xbsIndex_r4/Relational  mode=a=b  op_type=Bool  en=off  latency=0  dbl_ovrd=off  block_type=relational
  Relational1 : xbsIndex_r4/Relational  mode=a>=b  op_type=Bool  en=off  latency=0  dbl_ovrd=off  block_type=relational
  Relational2 : xbsIndex_r4/Relational  mode=a>b  op_type=Bool  en=off  latency=0  dbl_ovrd=off  block_type=relational
  Relational3 : xbsIndex_r4/Relational  mode=a!=b  op_type=Bool  en=off  latency=0  dbl_ovrd=off  block_type=relational
  Data Out : Outport  VectorParamsAs1DForOutWhenUnconnected=off
  Valid Out : Outport  Port=2  VectorParamsAs1DForOutWhenUnconnected=off
  Last Out : Outport  Port=3  VectorParamsAs1DForOutWhenUnconnected=off
  Size : Outport  Port=4  VectorParamsAs1DForOutWhenUnconnected=off
  Reset : Outport  Port=5  VectorParamsAs1DForOutWhenUnconnected=off
  wires:
  Register6/1 -> Size/1
  Logical2/1 -> Last Out/1, Reset/1, Counter1/1, Counter/1
  Relational1/1 -> Logical2/2
  Relational3/1 -> Logical2/1
  Constant1/1 -> Relational3/2
  Logical1/1 -> Register1/2
  Relational/1 -> Logical1/1
  Relational2/1 -> Logical/1
  Constant/1 -> Relational2/2, Relational/2
  Register5/1 -> Data Out/1
  Register4/1 -> Register5/1
  Register3/1 -> Valid Out/1
  Register2/1 -> Logical/2, Logical1/2
  Register1/1 -> Relational1/2, Relational3/1, Register6/1
  Counter1/1 -> Relational1/1
  Logical/1 -> Counter1/2, Register3/1
  Register/1 -> Register1/1, Register4/1
  Data In/1 -> Register/1
  Counter/1 -> Relational/1, Relational2/1
  Valid In/1 -> Counter/2, Register2/1

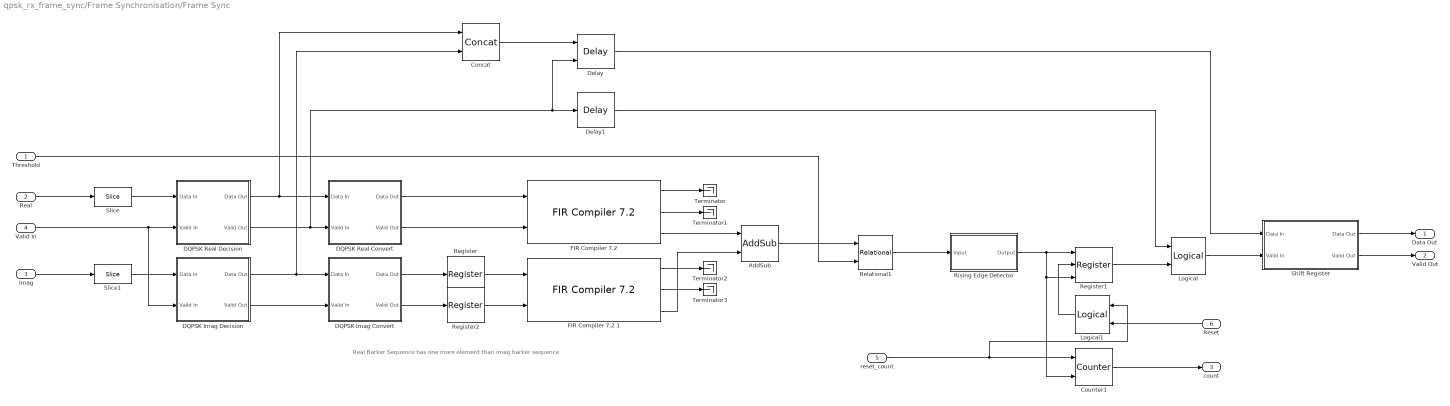
== system qpsk_rx_frame_sync/Frame Synchronisation/Frame Sync ==
  note: Real Barker Sequence has one more element than imag barker sequence
  Threshold : Inport
  Real : Inport  Port=2
  Imag : Inport  Port=3
  Valid In : Inport  Port=4
  reset_count : Inport  Port=5
  Reset : Inport  Port=6
  AddSub : xbsIndex_r4/AddSub  mode=Addition  use_carryin=off  use_carryout=off  en=off  latency=0  precision=Full  arith_type=Unsigned  n_bits=16  bin_pt=14  quantization=Truncate  overflow=Wrap  use_behavioral_HDL=off  hw_selection=Fabric  pipelined=off  dbl_ovrd=off  block_type=addsub
  Concat : xbsIndex_r4/Concat  num_inputs=2  dbl_ovrd=off  block_type=concat
  Counter1 : xbsIndex_r4/Counter  cnt_type=Free Running  cnt_to=Inf  operation=Up  start_count=0  cnt_by_val=1  arith_type=Unsigned  n_bits=32  bin_pt=0  load_pin=off  rst=on  en=on  explicit_period=off  period=1  use_behavioral_HDL=off  implementation=Fabric  dbl_ovrd=off  block_type=counter
  DQPSK Imag Convert : Subsystem
  DQPSK Imag Decision : Subsystem
  DQPSK Real Convert : Subsystem
  DQPSK Real Decision : Subsystem
  Delay : xbsIndex_r4/Delay  rst=off  infoeditControl=Selection of Reset will increase slice count due to use of real FFs and instead of SRLs  en=on  latency=3  reg_retiming=off  dbl_ovrd=off  block_type=delay
  Delay1 : xbsIndex_r4/Delay  rst=off  infoeditControl=Selection of Reset will increase slice count due to use of real FFs and instead of SRLs  en=off  latency=1  reg_retiming=off  dbl_ovrd=off  block_type=delay
  "FIR Compiler 7.2 " : xbsIndex_r4/FIR Compiler 7.2   coefficientvector=fliplr(double(fir_bbuf(1:2:end)))  coefficient_sets=1  coefficient_reload=off  filter_type=Single_Rate  rate_change_type=Integer  interpolation_rate=1  decimation_rate=1  zero_pack_factor=1  channel_sequence=Basic  number_channels=1  pattern_list='P4-0,P4-1,P4-2,P4-3,P4-4'  number_paths=1  ratespecification=Maximum_Possible  sampleperiod=20  hardwareoversamplingrate=1  coefficient_sign=Signed  quantization=Integer_Coefficients  coefficient_width=2  bestprecision=off  coefficient_fractional_bits=0  coefficient_structure=Inferred  output_rounding_mode=Full_Precision  output_width=21  filter_architecture=Systolic_Multiply_Accumulate  optimization_goal=Area  optimization_list='None'  data_buffer_type=Automatic  coefficient_buffer_type=Automatic  input_buffer_type=Automatic  output_buffer_type=Automatic  preference_for_other_storage=Automatic  multi_column_support=Automatic  columnconfig='20'  inter_column_pipe_length=4  data_has_tlast=Not_Required  m_data_has_tready=off  s_data_has_fifo=off  s_data_has_tuser=Not_Required  m_data_has_tuser=Not_Required  s_config_sync_mode=On_Vector  s_config_method=Single  num_reload_slots=1  has_aclken=on  has_aresetn=off  infoeditControl=ARESETn must be asserted for a minimum of 2 cycles  reset_data_vector=on  trim_axipin_name=on  simulation_type=hybrid_sim  simulation_model=sysgen:xfirv7_2_cmodel  data_path_portlist={ 's_axis_data_tdata', 'm_axis_data_tdata' }  passband_min=0.0  passband_max=0.5  stopband_min=0.5  stopband_max=1.0  filter_selection=1  gui_behaviour='Sysgen_GUI'  data_sign=Signed  data_width=16  data_fractional_bits=0  data_tuser_width=1  wrapper_available=true  ip_wrap_arbitrary_binary_point=true  ip_name=FIR Compiler  ip_version=7.2  dsptool_ready=true  ipcore_usecache=true  ipcore_useipmodelcache=true  port_translation_map={ 'aclken' => 'en', 'aresetn' => 'rst' }  run_core_at_system_period=true  ipcore_xco_need_fpga_part=true  block_type=fir_compiler_v7_2
      settings: infoedit=Maximum Possible : Maximizes oversampling rate. Abstracted input handshake (no s_data_tvalid) and automatic rate propagation.<br>Hardware Oversampling Rate : Specifies oversampling rate relative to the input sample period. Abstracted input handshake (no s_data_tvalid) and automatic rate propagation.<br>Input/Output Sample Period : Specifies absolute oversampling rate. No input handshake abstraction (exposes s_data_tvalid) and no rate propagation.
  FIR Compiler 7.2 1 : xbsIndex_r4/FIR Compiler 7.2   coefficientvector=fliplr(double(fir_bbuf(2:2:end)))  coefficient_sets=1  coefficient_reload=off  filter_type=Single_Rate  rate_change_type=Integer  interpolation_rate=1  decimation_rate=1  zero_pack_factor=1  channel_sequence=Basic  number_channels=1  pattern_list='P4-0,P4-1,P4-2,P4-3,P4-4'  number_paths=1  ratespecification=Maximum_Possible  sampleperiod=20  hardwareoversamplingrate=1  coefficient_sign=Signed  quantization=Integer_Coefficients  coefficient_width=2  bestprecision=off  coefficient_fractional_bits=0  coefficient_structure=Inferred  output_rounding_mode=Full_Precision  output_width=21  filter_architecture=Systolic_Multiply_Accumulate  optimization_goal=Area  optimization_list='None'  data_buffer_type=Automatic  coefficient_buffer_type=Automatic  input_buffer_type=Automatic  output_buffer_type=Automatic  preference_for_other_storage=Automatic  multi_column_support=Automatic  columnconfig='19'  inter_column_pipe_length=4  data_has_tlast=Not_Required  m_data_has_tready=off  s_data_has_fifo=off  s_data_has_tuser=Not_Required  m_data_has_tuser=Not_Required  s_config_sync_mode=On_Vector  s_config_method=Single  num_reload_slots=1  has_aclken=on  has_aresetn=off  infoeditControl=ARESETn must be asserted for a minimum of 2 cycles  reset_data_vector=on  trim_axipin_name=on  simulation_type=hybrid_sim  simulation_model=sysgen:xfirv7_2_cmodel  data_path_portlist={ 's_axis_data_tdata', 'm_axis_data_tdata' }  passband_min=0.0  passband_max=0.5  stopband_min=0.5  stopband_max=1.0  filter_selection=1  gui_behaviour='Sysgen_GUI'  data_sign=Signed  data_width=16  data_fractional_bits=0  data_tuser_width=1  wrapper_available=true  ip_wrap_arbitrary_binary_point=true  ip_name=FIR Compiler  ip_version=7.2  dsptool_ready=true  ipcore_usecache=true  ipcore_useipmodelcache=true  port_translation_map={ 'aclken' => 'en', 'aresetn' => 'rst' }  run_core_at_system_period=true  ipcore_xco_need_fpga_part=true  block_type=fir_compiler_v7_2
      settings: infoedit=Maximum Possible : Maximizes oversampling rate. Abstracted input handshake (no s_data_tvalid) and automatic rate propagation.<br>Hardware Oversampling Rate : Specifies oversampling rate relative to the input sample period. Abstracted input handshake (no s_data_tvalid) and automatic rate propagation.<br>Input/Output Sample Period : Specifies absolute oversampling rate. No input handshake abstraction (exposes s_data_tvalid) and no rate propagation.
  Logical : xbsIndex_r4/Logical  logical_function=AND  inputs=2  en=off  latency=0  precision=Full  arith_type=Unsigned  n_bits=16  bin_pt=0  align_bp=on  dbl_ovrd=off  block_type=logical
  Logical1 : xbsIndex_r4/Logical  logical_function=OR  inputs=2  en=off  latency=0  precision=Full  arith_type=Unsigned  n_bits=16  bin_pt=0  align_bp=on  dbl_ovrd=off  block_type=logical
  Register : xbsIndex_r4/Register  init=0  rst=off  en=off  dbl_ovrd=off  block_type=register
  Register1 : xbsIndex_r4/Register  init=0  rst=on  en=on  dbl_ovrd=off  block_type=register
  Register2 : xbsIndex_r4/Register  init=0  rst=off  en=off  dbl_ovrd=off  block_type=register
  Relational1 : xbsIndex_r4/Relational  mode=a>=b  op_type=Bool  en=off  latency=0  dbl_ovrd=off  block_type=relational
  Rising Edge Detector : Subsystem
  Shift Register : Subsystem
  Slice : xbsIndex_r4/Slice  nbits=1  boolean_output=off  mode=Upper Bit Location + Width  bit1=0  base1=MSB of Input  bit0=0  base0=LSB of Input  dbl_ovrd=off  block_type=slice
  Slice1 : xbsIndex_r4/Slice  nbits=1  boolean_output=off  mode=Upper Bit Location + Width  bit1=0  base1=MSB of Input  bit0=0  base0=LSB of Input  dbl_ovrd=off  block_type=slice
  Terminator{,1..3} (4 alike) : Terminator
  Data Out : Outport  VectorParamsAs1DForOutWhenUnconnected=off
  Valid Out : Outport  Port=2  VectorParamsAs1DForOutWhenUnconnected=off
  count : Outport  Port=3  VectorParamsAs1DForOutWhenUnconnected=off
  wires:
  Shift Register/2(Valid Out) -> Valid Out/1
  Real/1 -> Slice/1
  DQPSK Real Decision/2(Valid Out) -> Delay/2, Delay1/1, DQPSK Real Convert/2(Valid In)
  reset_count/1 -> Counter1/1, Logical1/1
  "FIR Compiler 7.2 "/1 -> Terminator/1
  DQPSK Real Convert/2(Valid Out) -> "FIR Compiler 7.2 "/2
  Shift Register/1(Data Out) -> Data Out/1
  Register1/1 -> Logical/2
  Rising Edge Detector/1(Output) -> Register1/1, Register1/3, Counter1/2
  "FIR Compiler 7.2 "/2 -> Terminator1/1
  Slice/1 -> DQPSK Real Decision/1(Data In)
  Valid In/1 -> DQPSK Imag Decision/2(Valid In), DQPSK Real Decision/2(Valid In)
  Counter1/1 -> count/1
  Logical1/1 -> Register1/2
  Threshold/1 -> Relational1/2
  Logical/1 -> Shift Register/2(Valid In)
  DQPSK Real Decision/1(Data Out) -> Concat/1, DQPSK Real Convert/1(Data In)
  Relational1/1 -> Rising Edge Detector/1(Input)
  Reset/1 -> Logical1/2
  DQPSK Real Convert/1(Data Out) -> "FIR Compiler 7.2 "/1
  Imag/1 -> Slice1/1
  Slice1/1 -> DQPSK Imag Decision/1(Data In)
  DQPSK Imag Decision/1(Data Out) -> Concat/2, DQPSK Imag Convert/1(Data In)
  DQPSK Imag Decision/2(Valid Out) -> DQPSK Imag Convert/2(Valid In)
  "FIR Compiler 7.2 "/3 -> AddSub/1
  AddSub/1 -> Relational1/1
  FIR Compiler 7.2 1/3 -> AddSub/2
  FIR Compiler 7.2 1/2 -> Terminator3/1
  FIR Compiler 7.2 1/1 -> Terminator2/1
  DQPSK Imag Convert/1(Data Out) -> Register/1
  DQPSK Imag Convert/2(Valid Out) -> Register2/1
  Register/1 -> FIR Compiler 7.2 1/1
  Register2/1 -> FIR Compiler 7.2 1/2
  Concat/1 -> Delay/1
  Delay/1 -> Shift Register/1(Data In)
  Delay1/1 -> Logical/1
